simulink model "Mains"  (Simulink 8.7)
settings: Solver=ode23tb  SolverMode=SingleTasking  StartTime=0.0  StopTime=tfinal  FixedStep=dt  MaxStep=Ts/2  RelTol=1e-6  AbsTol=1e-6
values from neighbouring files (symbols this model uses):
  Dm = 0    [Para_Motor.m]
  Jm = 0.0532    [Para_Motor.m]
  Ld = 2.7e-3    (= 0.0027)    [Para_Motor.m]
  Lq = Ld    (= 0.0027)    [Para_Motor.m]
  Ofq = Ofpm*3/2*K_3T2    [Para_Motor.m]
  p = 4    [Para_Motor.m]
  Qm0 = 0    [Para_Motor.m]
  Ra = 0.145    [Para_Motor.m]
undefined symbols (not defined in the file or in its folder): DiscIntNeverNeededParam, fw_downlimit, fw_ki, fw_kp, fw_uplimit, Igbt_max, Jo, K_2T3, K_3T2, Kaff, Kid, Kiq, Kpp, Kpv, KTo, Kvff, Ldo, Lqo, magnitude, Ofqo, Svm, Tid, Tiq, Tiv, Tload, Trmax, Tsf, Tsi, Tsp, Tsr, Tsv, Udm, Uidm, Uiqm, Upm, Uqm, Urm, v_sat_fw, VoltCom_sw, Wrmax
undefined symbols (not defined in the file): T_cic_r, T_lpf_fw_ud, T_lpf_fw_uq, T_lpf_r, Tf
libraries: simulink x2
CloseFcn:
  | ;slview('closediagram',bdroot);
settings Model: Creator=zwn  LastModifiedBy=googol
settings SolverCC: ZeroCrossControl=DisableAll
settings DataIOCC: LimitDataPoints=off  SignalLoggingSaveFormat=ModelDataLogs  SaveOutput=off  SaveTime=off
settings OptimizationCC: BooleanDataType=off  ExpressionDepthLimit=2147483647  InitFltsAndDblsToZero=on
settings DebuggingCC: SaveWithParameterizedLinksMsg=none  SignalResolutionControl=TryResolveAllWithWarning  MultiTaskDSMMsg=warning  MultiTaskCondExecSysMsg=none  FcnCallInpInsideContextMsg=UseLocalSettings  UnconnectedInputMsg=none  UnconnectedOutputMsg=none  UnconnectedLineMsg=none  StateNameClashWarn=warning
settings HardwareCC: TargetUnknown=on
settings RTWCC: TemplateMakefile=grt.tmf
settings GRTTargetCC: TargetFcnLib=ansi_tfl_tmw.mat  ModelReferenceCompliant=off  CombineOutputUpdateFcns=off  MatFileLogging=off  GRTInterface=on

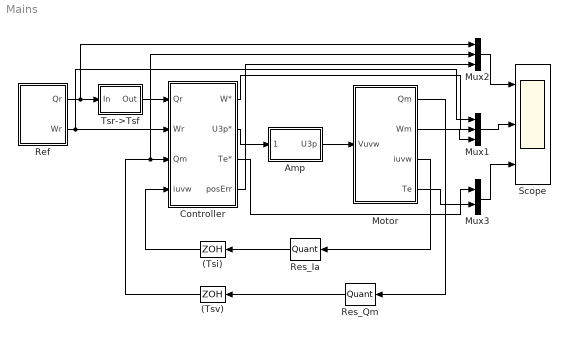
== system Mains ==
  (Tsi) : ZeroOrderHold  SampleTime=Tsi
  (Tsv) : ZeroOrderHold  SampleTime=Tsv
  Amp : Subsystem
  Controller : Subsystem
  Motor : Subsystem
  Mux1 : Mux  Inputs=3
  Mux2 : Mux  Inputs=3
  Mux3 : Mux  Inputs=2
  Ref : Subsystem
  Res_Ia : Quantizer  QuantizationInterval=Res_Ia
  Res_Qm : Quantizer  QuantizationInterval=Res_Qm
  Scope : Scope  NumInputPorts=3
  Tsr->Tsf : Subsystem
  wires:
  Motor/3(iuvw) -> Res_Ia/1
  (Tsi)/1 -> Controller/4(iuvw)
  Motor/1(Qm) -> Res_Qm/1
  (Tsv)/1 -> Controller/3(Qm), Mux2/2
  Mux1/1 -> Scope/2
  Res_Qm/1 -> (Tsv)/1
  Res_Ia/1 -> (Tsi)/1
  Ref/1(Qr) -> Tsr->Tsf/1(In), Mux2/1
  Tsr->Tsf/1(Out) -> Controller/1(Qr)
  Mux2/1 -> Scope/1
  Ref/2(Wr) -> Mux1/1, Controller/2(Wr)
  Mux3/1 -> Scope/3
  Motor/4(Te) -> Mux3/2
  Controller/3(Te*) -> Mux3/1
  Controller/2(U3p*) -> Amp/1(U3p*)
  Amp/1(U3p) -> Motor/1(Vuvw)
  Controller/4(posErr) -> Mux2/3
  Motor/2(Wm) -> Mux1/3
  Controller/1(W*) -> Mux1/2

== system Mains/Amp ==
  U3p* : Inport
  Constant2 : Constant  Value=[10 -5 -5]
  Manual Switch : ManualSwitch  CurrentSetting=0
  U3p : Outport
  wires:
  Constant2/1 -> Manual Switch/1
  Manual Switch/1 -> U3p/1
  U3p*/1 -> Manual Switch/2

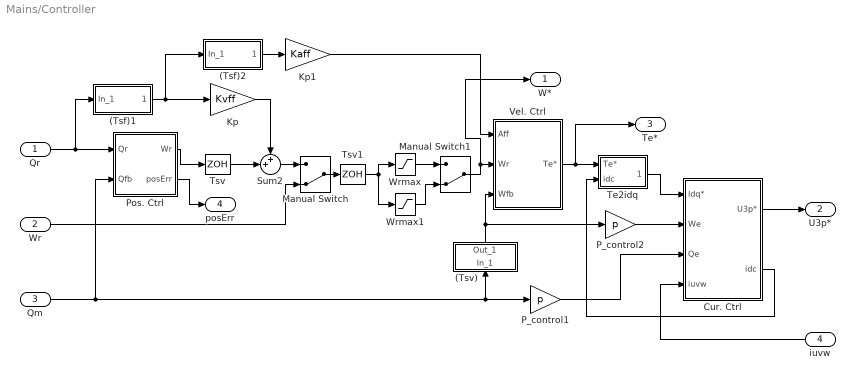
== system Mains/Controller ==
  Qr : Inport
  Wr : Inport  Port=2
  Qm : Inport  Port=3
  iuvw : Inport  Port=4
  (Tsf)1 : Subsystem  mask(Defference){Ts=Tsf, x0=0}
      mask prompts: Ts "Sample time Ts(s)"; x0 "Initial value x0"
      mask help: Enter expressions for a defference.
      mask Help: This block implements a defference. Unmask this block to see how it works. The defference term is implemented using a (1-z-1) block.
      mask Display: disp('(1-z-1)/Ts')
  (Tsf)2 : Subsystem  mask(Defference){Ts=Tsf, x0=0}
      mask prompts: Ts "Sample time Ts(s)"; x0 "Initial value x0"
      mask help: Enter expressions for a defference.
      mask Help: This block implements a defference. Unmask this block to see how it works. The defference term is implemented using a (1-z-1) block.
      mask Display: disp('(1-z-1)/Ts')
  (Tsv) : Subsystem  mask(Defference){Ts=Tsv, x0=Qm0}
      mask prompts: Ts "Sample time Ts(s)"; x0 "Initial value x0"
      mask help: Enter expressions for a defference.
      mask Help: This block implements a defference. Unmask this block to see how it works. The defference term is implemented using a (1-z-1) block.
      mask Display: disp('(1-z-1)/Ts')
  Cur. Ctrl : Subsystem
  Kp : Gain  Gain=Kvff  SaturateOnIntegerOverflow=on  OutDataTypeStr=Inherit: Same as input  ParamDataTypeStr=Inherit: Same as input
  Kp1 : Gain  Gain=Kaff  SaturateOnIntegerOverflow=on  OutDataTypeStr=Inherit: Same as input  ParamDataTypeStr=Inherit: Same as input
  Manual Switch : ManualSwitch  CurrentSetting=0
  Manual Switch1 : ManualSwitch  CurrentSetting=0
  P_control1 : Gain  Gain=p  SaturateOnIntegerOverflow=on  OutDataTypeStr=Inherit: Same as input  ParamDataTypeStr=Inherit: Same as input
  P_control2 : Gain  Gain=p  SaturateOnIntegerOverflow=on  OutDataTypeStr=Inherit: Same as input  ParamDataTypeStr=Inherit: Same as input
  Pos. Ctrl : Subsystem
  Sum2 : Sum  Inputs=++|  SampleTime=Tsp  SaturateOnIntegerOverflow=on  InputSameDT=on  OutDataTypeStr=Inherit: Same as first input
  Te2idq : Subsystem
  Tsv : ZeroOrderHold  SampleTime=Tsv
  Tsv1 : ZeroOrderHold  SampleTime=Tsv
  Vel. Ctrl : Subsystem
  Wrmax : Saturate  UpperLimit=Wrmax  LowerLimit=-Wrmax
  Wrmax1 : Saturate  UpperLimit=3*Wrmax  LowerLimit=-3*Wrmax
  W* : Outport
  U3p* : Outport  Port=2
  Te* : Outport  Port=3  InitialOutput=0
  posErr : Outport  Port=4
  wires:
  Qm/1 -> P_control1/1, (Tsv)/1(In_1), Pos. Ctrl/2(Qfb)
  P_control2/1 -> Cur. Ctrl/2(We)
  Vel. Ctrl/1(Te*) -> Te2idq/1(Te*), Te*/1
  Te2idq/1(Idq*) -> Cur. Ctrl/1(Idq*)
  (Tsv)/1(Out_1) -> Vel. Ctrl/3(Wfb), P_control2/1
  Cur. Ctrl/1(U3p*) -> U3p*/1
  P_control1/1 -> Cur. Ctrl/3(Qe)
  iuvw/1 -> Cur. Ctrl/4(iuvw)
  Pos. Ctrl/1(Wr) -> Tsv/1
  Qr/1 -> Pos. Ctrl/1(Qr), (Tsf)1/1(In_1)
  Tsv/1 -> Sum2/2
  (Tsf)1/1(Out_1) -> Kp/1, (Tsf)2/1(In_1)
  Kp/1 -> Sum2/1
  (Tsf)2/1(Out_1) -> Kp1/1
  Kp1/1 -> Vel. Ctrl/1(Aff)
  Sum2/1 -> Manual Switch/1
  Manual Switch/1 -> Tsv1/1
  Wr/1 -> Manual Switch/2
  Pos. Ctrl/2(posErr) -> posErr/1
  Cur. Ctrl/2(idc) -> Te2idq/2(idc)
  Wrmax/1 -> Manual Switch1/1
  Manual Switch1/1 -> W*/1, Vel. Ctrl/2(Wr)
  Wrmax1/1 -> Manual Switch1/2
  Tsv1/1 -> Wrmax/1, Wrmax1/1

== system Mains/Motor ==
  Vuvw : Inport
  Elec : Subsystem
  Mech : Subsystem
  Qm : Outport  InitialOutput=0
  Wm : Outport  Port=2  InitialOutput=0
  iuvw : Outport  Port=3  InitialOutput=0
  Te : Outport  Port=4  InitialOutput=0
  wires:
  Mech/2(Qm) -> Qm/1, Elec/3(Qm)
  Mech/1(Wm) -> Wm/1, Elec/2(Wm)
  Elec/1(iuvw) -> iuvw/1
  Elec/2(Te) -> Mech/1(Te), Te/1
  Vuvw/1 -> Elec/1(Vuvw)

== system Mains/Ref ==
  (T_cic_r,Tsr) : Subsystem  mask{n=round(T_cic_r/Tsr), Ts=Tsr}
      mask prompts: n "Steps"; Ts "Sampling time(s)"
      mask Display: disp('(1-z-n)/n(1-z-1)')
  1/s(Tsr) : DiscreteIntegrator  SampleTime=Tsr  UpperSaturationLimit=Trmax  LowerSaturationLimit=-Trmax  ICPrevOutput=DiscIntNeverNeededParam  ICPrevScaledInput=DiscIntNeverNeededParam
  Manual Switch : ManualSwitch
  Manual Switch1 : ManualSwitch
  Tf(Ts) : Subsystem  mask{Ts=Tsr, TL=T_lpf_r}
      mask prompts: Ts "Ts(s)"; TL "TL(s)"
      mask Display: disp('1/(1+TLs)')
  Wrr(rad/s) (Tsr) : FromWorkspace  VariableName=[twr,Wrr]  SampleTime=Tsr
  Qr : Outport
  Wr : Outport  Port=2
  wires:
  Wrr(rad/s) (Tsr)/1 -> (T_cic_r,Tsr)/1(In1), Manual Switch1/2, Tf(Ts)/1(In1)
  1/s(Tsr)/1 -> Qr/1
  Manual Switch/1 -> Wr/1, 1/s(Tsr)/1
  Tf(Ts)/1(Out1) -> Manual Switch/2
  Manual Switch1/1 -> Manual Switch/1
  (T_cic_r,Tsr)/1(Out1) -> Manual Switch1/1

== system Mains/Tsr->Tsf ==
  In : Inport
  Tsf : ZeroOrderHold  SampleTime=Tsf
  Tsr/Tsp(Tsf) : Subsystem  mask{n=round(Tsr/Tsf), Ts=Tsf}
      mask prompts: n "Sample number"; Ts "Sampling time(s)"
      mask Display: disp('CIC')
  Out : Outport
  wires:
  Tsf/1 -> Tsr/Tsp(Tsf)/1(In)
  In/1 -> Tsf/1
  Tsr/Tsp(Tsf)/1(Out) -> Out/1

== system Mains/Controller/(Tsf)1 ==
  In_1 : Inport
  Sum3 : Sum  Inputs=|+-  SaturateOnIntegerOverflow=on  InputSameDT=on  OutDataTypeStr=Inherit: Same as first input
  Ts(x0) : UnitDelay  InitialCondition=x0  SampleTime=Ts
  gear2 : Gain  Gain=1/Ts  SaturateOnIntegerOverflow=on  OutDataTypeStr=Inherit: Same as input  ParamDataTypeStr=Inherit: Same as input
  Out_1 : Outport  InitialOutput=0
  wires:
  In_1/1 -> Ts(x0)/1, Sum3/1
  Ts(x0)/1 -> Sum3/2
  Sum3/1 -> gear2/1
  gear2/1 -> Out_1/1

== system Mains/Controller/(Tsf)2 ==
  In_1 : Inport
  Sum3 : Sum  Inputs=|+-  SaturateOnIntegerOverflow=on  InputSameDT=on  OutDataTypeStr=Inherit: Same as first input
  Ts(x0) : UnitDelay  InitialCondition=x0  SampleTime=Ts
  gear2 : Gain  Gain=1/Ts  SaturateOnIntegerOverflow=on  OutDataTypeStr=Inherit: Same as input  ParamDataTypeStr=Inherit: Same as input
  Out_1 : Outport  InitialOutput=0
  wires:
  gear2/1 -> Out_1/1
  Sum3/1 -> gear2/1
  Ts(x0)/1 -> Sum3/2
  In_1/1 -> Sum3/1, Ts(x0)/1

== system Mains/Controller/(Tsv) ==
  In_1 : Inport
  Sum3 : Sum  Inputs=|+-  SaturateOnIntegerOverflow=on  InputSameDT=on  OutDataTypeStr=Inherit: Same as first input
  Ts(x0) : UnitDelay  InitialCondition=x0  SampleTime=Ts
  gear2 : Gain  Gain=1/Ts  SaturateOnIntegerOverflow=on  OutDataTypeStr=Inherit: Same as input  ParamDataTypeStr=Inherit: Same as input
  Out_1 : Outport  InitialOutput=0
  wires:
  gear2/1 -> Out_1/1
  Sum3/1 -> gear2/1
  Ts(x0)/1 -> Sum3/2
  In_1/1 -> Sum3/1, Ts(x0)/1

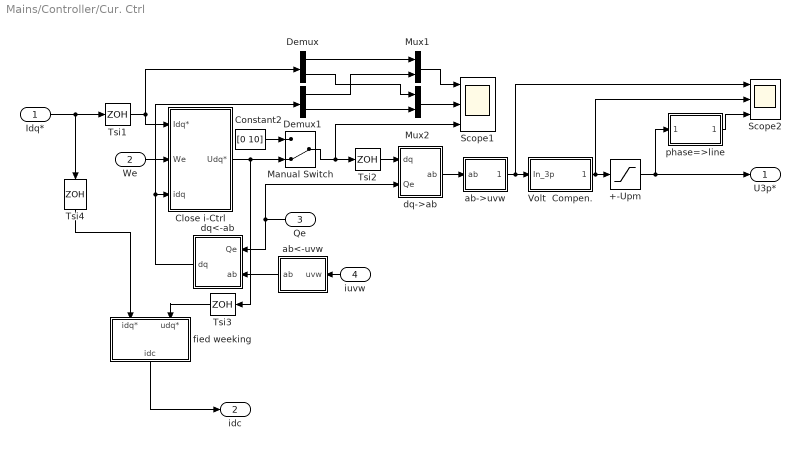
== system Mains/Controller/Cur. Ctrl ==
  Idq* : Inport
  We : Inport  Port=2
  Qe : Inport  Port=3
  iuvw : Inport  Port=4
  +-Upm : Saturate  UpperLimit=Upm  LowerLimit=-Upm
  Close i-Ctrl : Subsystem  TreatAsAtomicUnit=on
  Constant2 : Constant  Value=[0 10]
  Demux : Demux  Outputs=2
  Demux1 : Demux  Outputs=2
  Manual Switch : ManualSwitch  CurrentSetting=0
  Mux1 : Mux  Inputs=2
  Mux2 : Mux  Inputs=2
  Scope1 : Scope  NumInputPorts=3
  Scope2 : Scope  NumInputPorts=3
  Tsi{1..4} (4 alike) : ZeroOrderHold  SampleTime=Tsi
  Volt  Compen. : Subsystem
  ab->uvw : Subsystem
  ab<-uvw : Subsystem  TreatAsAtomicUnit=on
  dq->ab : Subsystem
  dq<-ab : Subsystem  TreatAsAtomicUnit=on
  fied weeking : Subsystem
  phase=>line : Subsystem
  U3p* : Outport
  idc : Outport  Port=2
  wires:
  Volt  Compen./1(Out_3p) -> +-Upm/1, Scope2/2
  dq->ab/1(ab) -> ab->uvw/1(ab)
  ab<-uvw/1(ab) -> dq<-ab/2(ab)
  iuvw/1 -> ab<-uvw/1(uvw)
  ab->uvw/1(uvw) -> Volt  Compen./1(In_3p), Scope2/1
  dq<-ab/1(dq) -> Close i-Ctrl/3(idq), Demux1/1
  Close i-Ctrl/1(Udq*) -> Tsi3/1, Manual Switch/2
  Manual Switch/1 -> Scope1/3, Tsi2/1
  Constant2/1 -> Manual Switch/1
  Qe/1 -> dq<-ab/1(Qe), dq->ab/2(Qe)
  Tsi1/1 -> Demux/1, Close i-Ctrl/1(Idq*)
  Mux1/1 -> Scope1/1
  Mux2/1 -> Scope1/2
  Demux/1 -> Mux1/1
  Demux1/1 -> Mux1/2
  Demux/2 -> Mux2/1
  Demux1/2 -> Mux2/2
  +-Upm/1 -> U3p*/1, phase=>line/1(U3p*)
  Idq*/1 -> Tsi4/1, Tsi1/1
  We/1 -> Close i-Ctrl/2(We)
  Tsi2/1 -> dq->ab/1(dq)
  phase=>line/1(U3l*) -> Scope2/3
  fied weeking/1(idc) -> idc/1
  Tsi3/1 -> fied weeking/2(udq*)
  Tsi4/1 -> fied weeking/1(idq*)

== system Mains/Controller/Pos. Ctrl ==
  Qr : Inport
  Qfb : Inport  Port=2
  Kp : Gain  Gain=Kpp  SaturateOnIntegerOverflow=on  OutDataTypeStr=Inherit: Same as input  ParamDataTypeStr=Inherit: Same as input
  Sum2 : Sum  Inputs=|+-  SampleTime=Tsp  SaturateOnIntegerOverflow=on  InputSameDT=on  OutDataTypeStr=Inherit: Same as first input
  Wr : Outport
  posErr : Outport  Port=2
  wires:
  Sum2/1 -> posErr/1, Kp/1
  Qfb/1 -> Sum2/2
  Qr/1 -> Sum2/1
  Kp/1 -> Wr/1

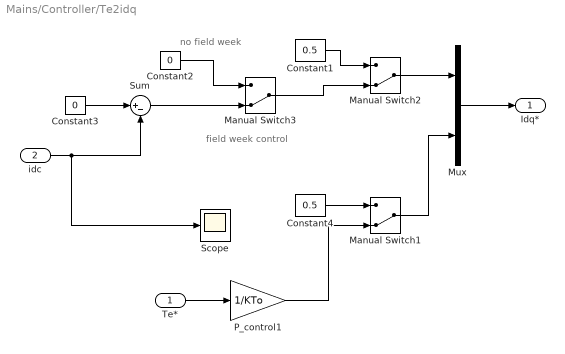
== system Mains/Controller/Te2idq ==
  note: field week control
  note: no field week
  Te* : Inport
  idc : Inport  Port=2
  Constant1 : Constant  Value=0.5
  Constant2 : Constant  Value=0
  Constant3 : Constant  Value=0
  Constant4 : Constant  Value=0.5
  Manual Switch1 : ManualSwitch  CurrentSetting=0
  Manual Switch2 : ManualSwitch  CurrentSetting=0
  Manual Switch3 : ManualSwitch  CurrentSetting=0
  Mux : Mux  Inputs=2
  P_control1 : Gain  Gain=1/KTo  SaturateOnIntegerOverflow=on  OutDataTypeStr=Inherit: Same as input  ParamDataTypeStr=Inherit: Same as input
  Scope : Scope
  Sum : Sum  Inputs=|+-
  Idq* : Outport
  wires:
  Te*/1 -> P_control1/1
  P_control1/1 -> Manual Switch1/2
  Constant1/1 -> Manual Switch2/1
  Manual Switch2/1 -> Mux/1
  Manual Switch1/1 -> Mux/2
  Mux/1 -> Idq*/1
  idc/1 -> Scope/1, Sum/2
  Constant3/1 -> Sum/1
  Sum/1 -> Manual Switch3/2
  Manual Switch3/1 -> Manual Switch2/2
  Constant2/1 -> Manual Switch3/1
  Constant4/1 -> Manual Switch1/1

== system Mains/Controller/Vel. Ctrl ==
  Aff : Inport
  Wr : Inport  Port=2
  Wfb : Inport  Port=3
  1/Ti : Gain  Gain=1/Tiv  SaturateOnIntegerOverflow=on  OutDataTypeStr=Inherit: Same as input  ParamDataTypeStr=Inherit: Same as input
  1/s : DiscreteIntegrator  SampleTime=Tsv  LimitOutput=on  UpperSaturationLimit=Svm  LowerSaturationLimit=-Svm  ICPrevOutput=DiscIntNeverNeededParam  ICPrevScaledInput=DiscIntNeverNeededParam
  P_control : Gain  Gain=Kpv  SaturateOnIntegerOverflow=on  OutDataTypeStr=Inherit: Same as input  ParamDataTypeStr=Inherit: Same as input
  P_control2 : Gain  Gain=Jo  SaturateOnIntegerOverflow=on  OutDataTypeStr=Inherit: Same as input  ParamDataTypeStr=Inherit: Same as input
  Sum : Sum  Inputs=+|+|+  SampleTime=Tsv  SaturateOnIntegerOverflow=on  InputSameDT=on  OutDataTypeStr=Inherit: Same as first input
  Sum1 : Sum  Inputs=|+-  SampleTime=Tsv  SaturateOnIntegerOverflow=on  InputSameDT=on  OutDataTypeStr=Inherit: Same as first input
  Tf(Ts) : Subsystem  mask{Ts=Tsv, TL=Tf}
      mask prompts: Ts "Ts(s)"; TL "TL(s)"
      mask Display: disp('1/(1+TLs)')
  Trmax : Saturate  UpperLimit=Trmax  LowerLimit=-Trmax
  Te* : Outport  InitialOutput=0
  wires:
  Sum/1 -> P_control2/1
  Sum1/1 -> P_control/1
  Wr/1 -> Sum1/1
  Wfb/1 -> Sum1/2
  Trmax/1 -> Tf(Ts)/1(In1)
  1/Ti/1 -> 1/s/1
  P_control/1 -> 1/Ti/1, Sum/3
  1/s/1 -> Sum/2
  Tf(Ts)/1(Out1) -> Te*/1
  P_control2/1 -> Trmax/1
  Aff/1 -> Sum/1

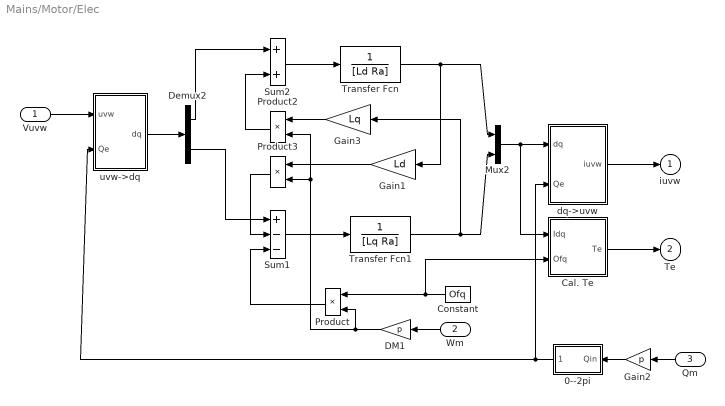
== system Mains/Motor/Elec ==
  Vuvw : Inport
  Wm : Inport  Port=2
  Qm : Inport  Port=3
  0--2pi : Subsystem
  Cal. Te : Subsystem
  Constant : Constant  Value=Ofq
  DM1 : Gain  Gain=p  SaturateOnIntegerOverflow=on  OutDataTypeStr=Inherit: Same as input  ParamDataTypeStr=Inherit: Same as input
  Demux2 : Demux  Outputs=2
  Gain1 : Gain  Gain=Ld  SaturateOnIntegerOverflow=on  OutDataTypeStr=Inherit: Same as input  ParamDataTypeStr=Inherit: Same as input
  Gain2 : Gain  Gain=p  SaturateOnIntegerOverflow=on  OutDataTypeStr=Inherit: Same as input  ParamDataTypeStr=Inherit: Same as input
  Gain3 : Gain  Gain=Lq  SaturateOnIntegerOverflow=on  OutDataTypeStr=Inherit: Same as input  ParamDataTypeStr=Inherit: Same as input
  Mux2 : Mux  Inputs=2
  Product : Product  SaturateOnIntegerOverflow=on  RndMeth=Zero  InputSameDT=on  OutDataTypeStr=Inherit: Same as first input
  Product2 : Product  SaturateOnIntegerOverflow=on  RndMeth=Zero  InputSameDT=on  OutDataTypeStr=Inherit: Same as first input
  Product3 : Product  SaturateOnIntegerOverflow=on  RndMeth=Zero  InputSameDT=on  OutDataTypeStr=Inherit: Same as first input
  Sum1 : Sum  Inputs=+--  SaturateOnIntegerOverflow=on  InputSameDT=on  OutDataTypeStr=Inherit: Same as first input
  Sum2 : Sum  SaturateOnIntegerOverflow=on  InputSameDT=on  OutDataTypeStr=Inherit: Same as first input
  Transfer Fcn : TransferFcn  Denominator=[Ld Ra]
  Transfer Fcn1 : TransferFcn  Denominator=[Lq Ra]
  dq->uvw : Subsystem
  uvw->dq : Subsystem
  iuvw : Outport  InitialOutput=0
  Te : Outport  Port=2  InitialOutput=0
  wires:
  0--2pi/1(Qout) -> dq->uvw/2(Qe), uvw->dq/2(Qe)
  Product/1 -> Sum1/3
  Constant/1 -> Product/1, Cal. Te/2(Ofq)
  Mux2/1 -> dq->uvw/1(dq), Cal. Te/1(Idq)
  dq->uvw/1(iuvw) -> iuvw/1
  DM1/1 -> Product/2, Product3/2, Product2/2
  Wm/1 -> DM1/1
  Product2/1 -> Sum2/2
  Product3/1 -> Sum1/2
  Gain1/1 -> Product3/1
  Gain3/1 -> Product2/1
  Demux2/2 -> Sum1/1
  Transfer Fcn/1 -> Mux2/1, Gain1/1
  Transfer Fcn1/1 -> Mux2/2, Gain3/1
  Sum1/1 -> Transfer Fcn1/1
  Demux2/1 -> Sum2/1
  uvw->dq/1(dq) -> Demux2/1
  Sum2/1 -> Transfer Fcn/1
  Qm/1 -> Gain2/1
  Gain2/1 -> 0--2pi/1(Qin)
  Vuvw/1 -> uvw->dq/1(uvw)
  Cal. Te/1(Te) -> Te/1

== system Mains/Motor/Mech ==
  Te : Inport
  1/JM : Gain  Gain=1/Jm  SaturateOnIntegerOverflow=on  OutDataTypeStr=Inherit: Same as input  ParamDataTypeStr=Inherit: Same as input
  Constant2 : Constant  Value=Tload
  DM : Gain  Gain=Dm  SaturateOnIntegerOverflow=on  OutDataTypeStr=Inherit: Same as input  ParamDataTypeStr=Inherit: Same as input
  Qm0 : Integrator  InitialCondition=Qm0
  Sum1 : Sum  Inputs=-|+|-  SaturateOnIntegerOverflow=on  InputSameDT=on  OutDataTypeStr=Inherit: Same as first input
  velocity4 : Integrator
  Wm : Outport  InitialOutput=0
  Qm : Outport  Port=2  InitialOutput=0
  wires:
  1/JM/1 -> velocity4/1
  Qm0/1 -> Qm/1
  velocity4/1 -> Qm0/1, DM/1, Wm/1
  Te/1 -> Sum1/2
  Sum1/1 -> 1/JM/1
  Constant2/1 -> Sum1/3
  DM/1 -> Sum1/1

== system Mains/Ref/(T_cic_r,Tsr) ==
  In1 : Inport
  (1/z)^n : DiscreteTransferFcn  Denominator=[1 zeros(1,n)]  SampleTime=Ts
  1/z(Ts) : UnitDelay  SampleTime=Ts
  Sum3 : Sum  Inputs=-+|  SaturateOnIntegerOverflow=on  InputSameDT=on  OutDataTypeStr=Inherit: Same as first input
  Sum4 : Sum  Inputs=|++  SaturateOnIntegerOverflow=on  InputSameDT=on  OutDataTypeStr=Inherit: Same as first input
  pMum : Gain  Gain=1/n  SaturateOnIntegerOverflow=on  OutDataTypeStr=Inherit: Same as input  ParamDataTypeStr=Inherit: Same as input
  Out1 : Outport
  wires:
  pMum/1 -> Sum4/1
  Sum4/1 -> 1/z(Ts)/1, Out1/1
  1/z(Ts)/1 -> Sum4/2
  Sum3/1 -> pMum/1
  (1/z)^n/1 -> Sum3/1
  In1/1 -> (1/z)^n/1, Sum3/2

== system Mains/Ref/Tf(Ts) ==
  In1 : Inport
  LPF : DiscreteFilter  Numerator=[Ts/(Ts+TL)]  Denominator=[1 -(1-Ts/(Ts+TL))]  SampleTime=Ts
  Out1 : Outport
  wires:
  LPF/1 -> Out1/1
  In1/1 -> LPF/1

== system Mains/Tsr->Tsf/Tsr/Tsp(Tsf) ==
  In : Inport
  (1/z)^n : DiscreteTransferFcn  Denominator=[1 zeros(1,n)]  SampleTime=Ts
  1/z(Ts) : UnitDelay  SampleTime=Ts
  Sum3 : Sum  Inputs=-+|  SampleTime=Ts  SaturateOnIntegerOverflow=on  InputSameDT=on  OutDataTypeStr=Inherit: Same as first input
  Sum4 : Sum  Inputs=|++  SaturateOnIntegerOverflow=on  InputSameDT=on  OutDataTypeStr=Inherit: Same as first input
  pMum : Gain  Gain=1/n  SaturateOnIntegerOverflow=on  OutDataTypeStr=Inherit: Same as input  ParamDataTypeStr=Inherit: Same as input
  Out : Outport
  wires:
  In/1 -> Sum3/2, (1/z)^n/1
  (1/z)^n/1 -> Sum3/1
  Sum3/1 -> Sum4/1
  1/z(Ts)/1 -> Sum4/2
  Sum4/1 -> 1/z(Ts)/1, pMum/1
  pMum/1 -> Out/1

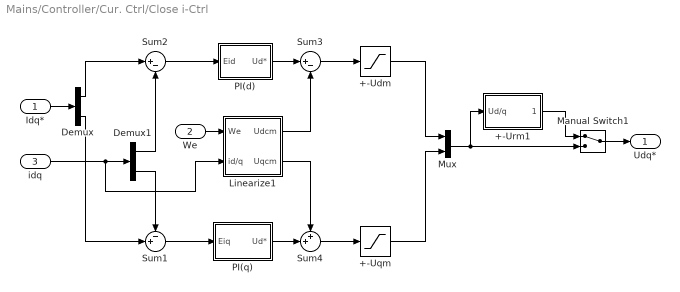
== system Mains/Controller/Cur. Ctrl/Close i-Ctrl ==
  Idq* : Inport
  We : Inport  Port=2
  idq : Inport  Port=3
  +-Udm : Saturate  UpperLimit=Udm  LowerLimit=-Udm
  +-Uqm : Saturate  UpperLimit=Uqm  LowerLimit=-Uqm
  +-Urm1 : Subsystem
  Demux : Demux  Outputs=2
  Demux1 : Demux  Outputs=2
  Linearize1 : Subsystem  TreatAsAtomicUnit=on
  Manual Switch1 : ManualSwitch
  Mux : Mux  Inputs=2
  PI(d) : Subsystem
  PI(q) : Subsystem
  Sum1 : Sum  Inputs=-+|  SaturateOnIntegerOverflow=on  InputSameDT=on  OutDataTypeStr=Inherit: Same as first input
  Sum2 : Sum  Inputs=|+-  SaturateOnIntegerOverflow=on  InputSameDT=on  OutDataTypeStr=Inherit: Same as first input
  Sum3 : Sum  Inputs=|+-  SaturateOnIntegerOverflow=on  InputSameDT=on  OutDataTypeStr=Inherit: Same as first input
  Sum4 : Sum  Inputs=++|  SaturateOnIntegerOverflow=on  InputSameDT=on  OutDataTypeStr=Inherit: Same as first input
  Udq* : Outport
  wires:
  idq/1 -> Linearize1/2(id/q), Demux1/1
  We/1 -> Linearize1/1(We)
  Sum4/1 -> +-Uqm/1
  Sum3/1 -> +-Udm/1
  PI(q)/1(Ud*) -> Sum4/2
  Demux1/1 -> Sum2/2
  Demux1/2 -> Sum1/1
  Sum2/1 -> PI(d)/1(Eid)
  PI(d)/1(Ud*) -> Sum3/1
  Sum1/1 -> PI(q)/1(Eiq)
  +-Udm/1 -> Mux/1
  +-Uqm/1 -> Mux/2
  Demux/1 -> Sum2/1
  Idq*/1 -> Demux/1
  Demux/2 -> Sum1/2
  Linearize1/1(Udcm) -> Sum3/2
  Linearize1/2(Uqcm) -> Sum4/1
  Manual Switch1/1 -> Udq*/1
  Mux/1 -> Manual Switch1/2, +-Urm1/1(Ud/q)
  +-Urm1/1(Ud/qO) -> Manual Switch1/1

== system Mains/Controller/Cur. Ctrl/Volt  Compen. ==
  In_3p : Inport
  Constant : Constant  Value=VoltCom_sw
  Constant1 : Constant  Value=0
  Multiport Switch : MultiPortSwitch  SampleTime=Tsi  SaturateOnIntegerOverflow=on  InputSameDT=on
  Sum3 : Sum  SaturateOnIntegerOverflow=on  InputSameDT=on  OutDataTypeStr=Inherit: Same as first input
  Volt Compen 1 : Subsystem
  Volt Compen 2 : Subsystem
  Out_3p : Outport
  wires:
  In_3p/1 -> Volt Compen 1/1(Uuvw), Volt Compen 2/1(Uuvw), Sum3/1
  Multiport Switch/1 -> Sum3/2
  Constant1/1 -> Multiport Switch/4
  Constant/1 -> Multiport Switch/1
  Volt Compen 2/1(Uh2) -> Multiport Switch/3
  Volt Compen 1/1(Uh1) -> Multiport Switch/2
  Sum3/1 -> Out_3p/1

== system Mains/Controller/Cur. Ctrl/ab->uvw ==
  ab : Inport
  Constant1 : Constant  Value=[-1/2 sqrt(3)/2]  SampleTime=Tsi
  Constant2 : Constant  Value=[1 0]  SampleTime=Tsi
  Constant3 : Constant  Value=[-1/2 -sqrt(3)/2]  SampleTime=Tsi
  Dot Product : DotProduct  InputSameDT=on  OutDataTypeStr=Inherit: Inherit via internal rule
  Dot Product1 : DotProduct  InputSameDT=on  OutDataTypeStr=Inherit: Inherit via internal rule
  Dot Product2 : DotProduct  InputSameDT=on  OutDataTypeStr=Inherit: Inherit via internal rule
  Gain5 : Gain  Gain=K_2T3  SaturateOnIntegerOverflow=on  OutDataTypeStr=Inherit: Same as input  ParamDataTypeStr=Inherit: Same as input
  Mux1 : Mux  Inputs=3
  uvw : Outport  InitialOutput=0
  wires:
  Dot Product1/1 -> Mux1/2
  Dot Product/1 -> Mux1/1
  Constant2/1 -> Dot Product/2
  Constant1/1 -> Dot Product1/2
  ab/1 -> Dot Product/1, Dot Product1/1, Dot Product2/1
  Mux1/1 -> Gain5/1
  Constant3/1 -> Dot Product2/2
  Dot Product2/1 -> Mux1/3
  Gain5/1 -> uvw/1

== system Mains/Controller/Cur. Ctrl/ab<-uvw ==
  uvw : Inport
  Constant1 : Constant  Value=[0 1 -1]*sqrt(3)/2  SampleTime=Tsi
  Constant2 : Constant  Value=[1 -0.5 -0.5]  SampleTime=Tsi
  Dot Product : DotProduct  InputSameDT=on  OutDataTypeStr=Inherit: Inherit via internal rule
  Dot Product1 : DotProduct  InputSameDT=on  OutDataTypeStr=Inherit: Inherit via internal rule
  Gain5 : Gain  Gain=K_3T2  SaturateOnIntegerOverflow=on  OutDataTypeStr=Inherit: Same as input  ParamDataTypeStr=Inherit: Same as input
  Mux1 : Mux  Inputs=2
  ab : Outport  InitialOutput=0
  wires:
  Dot Product1/1 -> Mux1/2
  Constant1/1 -> Dot Product1/2
  Dot Product/1 -> Mux1/1
  uvw/1 -> Dot Product1/1, Dot Product/1
  Constant2/1 -> Dot Product/2
  Gain5/1 -> ab/1
  Mux1/1 -> Gain5/1

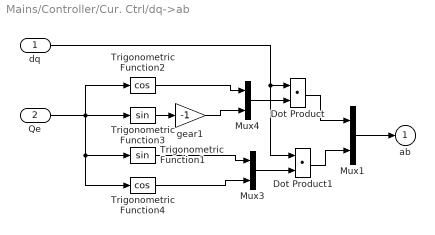
== system Mains/Controller/Cur. Ctrl/dq->ab ==
  dq : Inport
  Qe : Inport  Port=2
  Dot Product : DotProduct  InputSameDT=on  OutDataTypeStr=Inherit: Inherit via internal rule
  Dot Product1 : DotProduct  InputSameDT=on  OutDataTypeStr=Inherit: Inherit via internal rule
  Mux1 : Mux  Inputs=2
  Mux3 : Mux  Inputs=2
  Mux4 : Mux  Inputs=2
  Trigonometric Function1 : Trigonometry
  Trigonometric Function2 : Trigonometry  Operator=cos
  Trigonometric Function3 : Trigonometry
  Trigonometric Function4 : Trigonometry  Operator=cos
  gear1 : Gain  Gain=-1  SaturateOnIntegerOverflow=on  OutDataTypeStr=Inherit: Same as input  ParamDataTypeStr=Inherit: Same as input
  ab : Outport  InitialOutput=0
  wires:
  Mux1/1 -> ab/1
  dq/1 -> Dot Product/1, Dot Product1/1
  Qe/1 -> Trigonometric Function3/1, Trigonometric Function2/1, Trigonometric Function1/1, Trigonometric Function4/1
  Trigonometric Function1/1 -> Mux3/1
  Trigonometric Function4/1 -> Mux3/2
  Trigonometric Function2/1 -> Mux4/1
  Trigonometric Function3/1 -> gear1/1
  Mux3/1 -> Dot Product1/2
  Mux4/1 -> Dot Product/2
  Dot Product1/1 -> Mux1/2
  Dot Product/1 -> Mux1/1
  gear1/1 -> Mux4/2

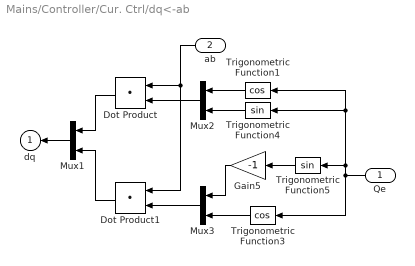
== system Mains/Controller/Cur. Ctrl/dq<-ab ==
  Qe : Inport
  ab : Inport  Port=2
  Dot Product : DotProduct  InputSameDT=on  OutDataTypeStr=Inherit: Inherit via internal rule
  Dot Product1 : DotProduct  InputSameDT=on  OutDataTypeStr=Inherit: Inherit via internal rule
  Gain5 : Gain  Gain=-1  SaturateOnIntegerOverflow=on  OutDataTypeStr=Inherit: Same as input  ParamDataTypeStr=Inherit: Same as input
  Mux1 : Mux  Inputs=2
  Mux2 : Mux  Inputs=2
  Mux3 : Mux  Inputs=2
  Trigonometric Function1 : Trigonometry  Operator=cos
  Trigonometric Function3 : Trigonometry  Operator=cos
  Trigonometric Function4 : Trigonometry
  Trigonometric Function5 : Trigonometry
  dq : Outport  InitialOutput=0
  wires:
  Dot Product1/1 -> Mux1/2
  Mux3/1 -> Dot Product1/2
  Dot Product/1 -> Mux1/1
  ab/1 -> Dot Product1/1, Dot Product/1
  Mux2/1 -> Dot Product/2
  Trigonometric Function1/1 -> Mux2/1
  Mux1/1 -> dq/1
  Trigonometric Function4/1 -> Mux2/2
  Trigonometric Function3/1 -> Mux3/2
  Trigonometric Function5/1 -> Gain5/1
  Qe/1 -> Trigonometric Function1/1, Trigonometric Function4/1, Trigonometric Function5/1, Trigonometric Function3/1
  Gain5/1 -> Mux3/1

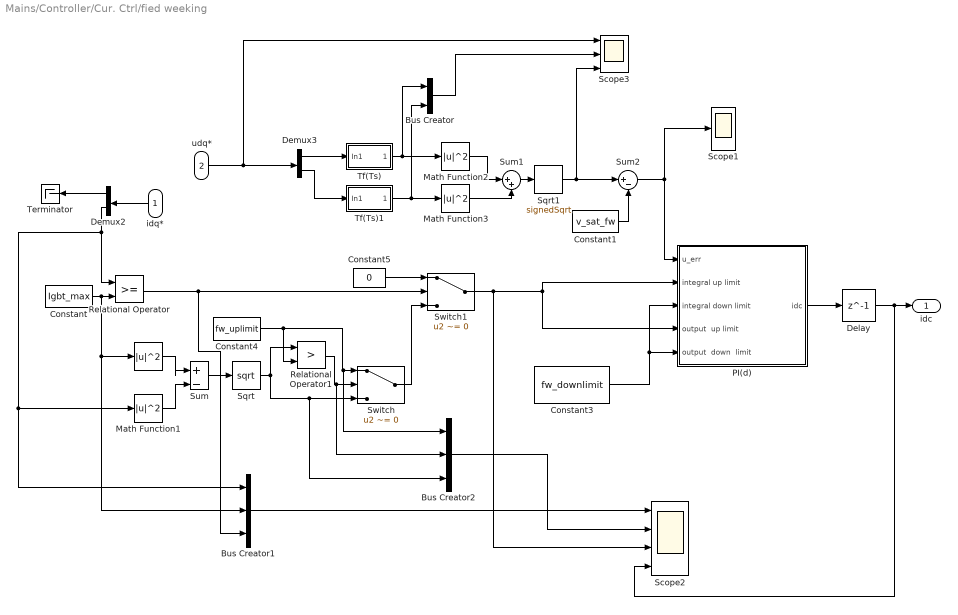
== system Mains/Controller/Cur. Ctrl/fied weeking ==
  idq* : Inport
  udq* : Inport  Port=2
  " " : Math  Operator=magnitude^2  SaturateOnIntegerOverflow=on
  Bus Creator : BusCreator  Inputs=2
  Bus Creator1 : BusCreator  Inputs=3
  Bus Creator2 : BusCreator  Inputs=3
  Constant : Constant  Value=Igbt_max
  Constant1 : Constant  Value=v_sat_fw
  Constant3 : Constant  Value=fw_downlimit
  Constant4 : Constant  Value=fw_uplimit
  Constant5 : Constant  Value=0
  Delay : Delay  DelayLength=1  SampleTime=Tsi
  Demux2 : Demux  Outputs=2
  Demux3 : Demux  Outputs=2
  Math Function1 : Math  Operator=magnitude^2  SaturateOnIntegerOverflow=on
  Math Function2 : Math  Operator=magnitude^2  OutputSignalType=real  SaturateOnIntegerOverflow=on
  Math Function3 : Math  Operator=magnitude^2  OutputSignalType=real  SaturateOnIntegerOverflow=on
  PI(d) : Subsystem
  Relational Operator : RelationalOperator  InputSameDT=on
  Relational Operator1 : RelationalOperator  Operator=>  InputSameDT=on
  Scope1 : Scope
  Scope2 : Scope  NumInputPorts=4
  Scope3 : Scope  NumInputPorts=3
  Sqrt : Sqrt  SaturateOnIntegerOverflow=on
  Sqrt1 : Sqrt  Operator=signedSqrt  OutputSignalType=real  SaturateOnIntegerOverflow=on
  Sum : Sum  Inputs=|+-
  Sum1 : Sum  Inputs=|++
  Sum2 : Sum  Inputs=|+-
  Switch : Switch  Criteria=u2 ~= 0
  Switch1 : Switch  Criteria=u2 ~= 0
  Terminator : Terminator
  Tf(Ts) : Subsystem  mask{Ts=Tsi, TL=T_lpf_fw_ud}
      mask prompts: Ts "Ts(s)"; TL "TL(s)"
      mask Display: disp('1/(1+TLs)')
  Tf(Ts)1 : Subsystem  mask{Ts=Tsi, TL=T_lpf_fw_uq}
      mask prompts: Ts "Ts(s)"; TL "TL(s)"
      mask Display: disp('1/(1+TLs)')
  idc : Outport
  wires:
  Demux2/2 -> Bus Creator1/1, Math Function1/1, Relational Operator/1
  Demux2/1 -> Terminator/1
  Relational Operator1/1 -> Bus Creator2/2, Switch/2
  Constant/1 -> Bus Creator1/2, " "/1, Relational Operator/2
  PI(d)/1(idc) -> Delay/1
  Switch/1 -> Switch1/3
  Constant5/1 -> Switch1/1
  Switch1/1 -> PI(d)/2(integral up limit), PI(d)/4(output  up limit), Scope2/3
  Tf(Ts)/1(Out1) -> Bus Creator/1, Math Function2/1
  Tf(Ts)1/1(Out1) -> Bus Creator/2, Math Function3/1
  Sum/1 -> Sqrt/1
  Constant3/1 -> PI(d)/3(integral down limit), PI(d)/5(output  down  limit)
  Relational Operator/1 -> Bus Creator1/3, Switch1/2
  " "/1 -> Sum/1
  Math Function1/1 -> Sum/2
  Constant1/1 -> Sum2/2
  Math Function3/1 -> Sum1/2
  udq*/1 -> Scope3/1, Demux3/1
  Sum1/1 -> Sqrt1/1
  Demux3/1 -> Tf(Ts)/1(In1)
  idq*/1 -> Demux2/1
  Demux3/2 -> Tf(Ts)1/1(In1)
  Math Function2/1 -> Sum1/1
  Sqrt1/1 -> Scope3/3, Sum2/1
  Constant4/1 -> Bus Creator2/1, Switch/1, Relational Operator1/2
  Sum2/1 -> Scope1/1, PI(d)/1(u_err)
  Sqrt/1 -> Relational Operator1/1, Bus Creator2/3, Switch/3
  Delay/1 -> Scope2/4, idc/1
  Bus Creator/1 -> Scope3/2
  Bus Creator1/1 -> Scope2/1
  Bus Creator2/1 -> Scope2/2

== system Mains/Controller/Cur. Ctrl/phase=>line ==
  U3p* : Inport
  Demux2 : Demux  Outputs=3
  Mux3 : Mux  Inputs=3
  Sum1 : Sum  Inputs=|+-  SaturateOnIntegerOverflow=on  InputSameDT=on  OutDataTypeStr=Inherit: Same as first input
  Sum2 : Sum  Inputs=|+-  SaturateOnIntegerOverflow=on  InputSameDT=on  OutDataTypeStr=Inherit: Same as first input
  Sum3 : Sum  Inputs=|+-  SaturateOnIntegerOverflow=on  InputSameDT=on  OutDataTypeStr=Inherit: Same as first input
  U3l* : Outport
  wires:
  Demux2/1 -> Sum2/1, Sum3/2
  Demux2/2 -> Sum1/1, Sum2/2
  Demux2/3 -> Sum3/1, Sum1/2
  Sum2/1 -> Mux3/1
  Sum1/1 -> Mux3/2
  Sum3/1 -> Mux3/3
  U3p*/1 -> Demux2/1
  Mux3/1 -> U3l*/1

== system Mains/Controller/Vel. Ctrl/Tf(Ts) ==
  In1 : Inport
  LPF : DiscreteFilter  Numerator=[Ts/(Ts+TL)]  Denominator=[1 -(1-Ts/(Ts+TL))]  SampleTime=Ts
  Out1 : Outport
  wires:
  LPF/1 -> Out1/1
  In1/1 -> LPF/1

== system Mains/Motor/Elec/0--2pi ==
  Qin : Inport
  Rounding Function : Rounding
  Sum2 : Sum  Inputs=|+-  SaturateOnIntegerOverflow=on  InputSameDT=on  OutDataTypeStr=Inherit: Same as first input
  ki1 : Gain  Gain=1/2/pi  SaturateOnIntegerOverflow=on  OutDataTypeStr=Inherit: Same as input  ParamDataTypeStr=Inherit: Same as input
  ki3 : Gain  Gain=2*pi  SaturateOnIntegerOverflow=on  OutDataTypeStr=Inherit: Same as input  ParamDataTypeStr=Inherit: Same as input
  Qout : Outport  InitialOutput=0
  wires:
  Qin/1 -> ki1/1
  ki3/1 -> Qout/1
  Sum2/1 -> ki3/1
  ki1/1 -> Sum2/1, Rounding Function/1
  Rounding Function/1 -> Sum2/2

== system Mains/Motor/Elec/Cal. Te ==
  Idq : Inport
  Ofq : Inport  Port=2
  DM : Gain  Gain=p  SaturateOnIntegerOverflow=on  OutDataTypeStr=Inherit: Same as input  ParamDataTypeStr=Inherit: Same as input
  Demux : Demux  Outputs=2
  Gain4 : Gain  Gain=Ld-Lq  SaturateOnIntegerOverflow=on  OutDataTypeStr=Inherit: Same as input  ParamDataTypeStr=Inherit: Same as input
  Product2 : Product  SaturateOnIntegerOverflow=on  RndMeth=Zero  InputSameDT=on  OutDataTypeStr=Inherit: Same as first input
  Sum2 : Sum  Inputs=++|  SampleTime=Tsp  SaturateOnIntegerOverflow=on  InputSameDT=on  OutDataTypeStr=Inherit: Same as first input
  Te : Outport
  wires:
  Idq/1 -> Demux/1
  Demux/1 -> Gain4/1
  DM/1 -> Te/1
  Gain4/1 -> Sum2/2
  Ofq/1 -> Sum2/1
  Sum2/1 -> Product2/1
  Demux/2 -> Product2/2
  Product2/1 -> DM/1

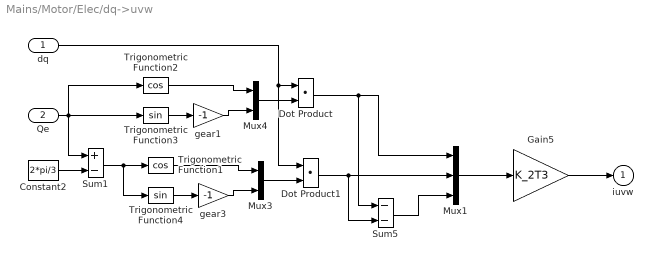
== system Mains/Motor/Elec/dq->uvw ==
  dq : Inport
  Qe : Inport  Port=2
  Constant2 : Constant  Value=2*pi/3
  Dot Product : DotProduct  InputSameDT=on  OutDataTypeStr=Inherit: Inherit via internal rule
  Dot Product1 : DotProduct  InputSameDT=on  OutDataTypeStr=Inherit: Inherit via internal rule
  Gain5 : Gain  Gain=K_2T3  SaturateOnIntegerOverflow=on  OutDataTypeStr=Inherit: Same as input  ParamDataTypeStr=Inherit: Same as input
  Mux1 : Mux  Inputs=3
  Mux3 : Mux  Inputs=2
  Mux4 : Mux  Inputs=2
  Sum1 : Sum  Inputs=+-  SaturateOnIntegerOverflow=on  InputSameDT=on  OutDataTypeStr=Inherit: Same as first input
  Sum5 : Sum  Inputs=--  SaturateOnIntegerOverflow=on  InputSameDT=on  OutDataTypeStr=Inherit: Same as first input
  Trigonometric Function1 : Trigonometry  Operator=cos
  Trigonometric Function2 : Trigonometry  Operator=cos
  Trigonometric Function3 : Trigonometry
  Trigonometric Function4 : Trigonometry
  gear1 : Gain  Gain=-1  SaturateOnIntegerOverflow=on  OutDataTypeStr=Inherit: Same as input  ParamDataTypeStr=Inherit: Same as input
  gear3 : Gain  Gain=-1  SaturateOnIntegerOverflow=on  OutDataTypeStr=Inherit: Same as input  ParamDataTypeStr=Inherit: Same as input
  iuvw : Outport  InitialOutput=0
  wires:
  Mux1/1 -> Gain5/1
  dq/1 -> Dot Product/1, Dot Product1/1
  Constant2/1 -> Sum1/2
  Qe/1 -> Sum1/1, Trigonometric Function3/1, Trigonometric Function2/1
  Sum1/1 -> Trigonometric Function1/1, Trigonometric Function4/1
  Trigonometric Function1/1 -> Mux3/1
  Trigonometric Function4/1 -> gear3/1
  gear3/1 -> Mux3/2
  Trigonometric Function2/1 -> Mux4/1
  Trigonometric Function3/1 -> gear1/1
  gear1/1 -> Mux4/2
  Mux3/1 -> Dot Product1/2
  Mux4/1 -> Dot Product/2
  Dot Product/1 -> Mux1/1, Sum5/1
  Dot Product1/1 -> Mux1/2, Sum5/2
  Sum5/1 -> Mux1/3
  Gain5/1 -> iuvw/1

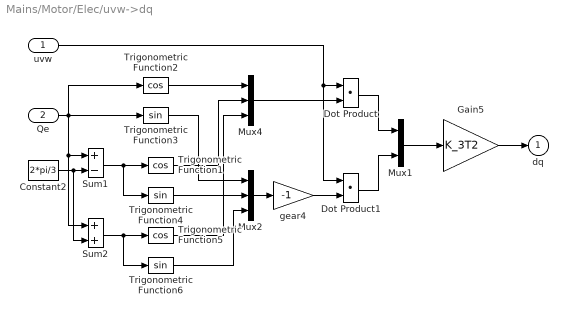
== system Mains/Motor/Elec/uvw->dq ==
  uvw : Inport
  Qe : Inport  Port=2
  Constant2 : Constant  Value=2*pi/3
  Dot Product : DotProduct  InputSameDT=on  OutDataTypeStr=Inherit: Inherit via internal rule
  Dot Product1 : DotProduct  InputSameDT=on  OutDataTypeStr=Inherit: Inherit via internal rule
  Gain5 : Gain  Gain=K_3T2  SaturateOnIntegerOverflow=on  OutDataTypeStr=Inherit: Same as input  ParamDataTypeStr=Inherit: Same as input
  Mux1 : Mux  Inputs=2
  Mux2 : Mux  Inputs=3
  Mux4 : Mux  Inputs=3
  Sum1 : Sum  Inputs=+-  SaturateOnIntegerOverflow=on  InputSameDT=on  OutDataTypeStr=Inherit: Same as first input
  Sum2 : Sum  SaturateOnIntegerOverflow=on  InputSameDT=on  OutDataTypeStr=Inherit: Same as first input
  Trigonometric Function1 : Trigonometry  Operator=cos
  Trigonometric Function2 : Trigonometry  Operator=cos
  Trigonometric Function3 : Trigonometry
  Trigonometric Function4 : Trigonometry
  Trigonometric Function5 : Trigonometry  Operator=cos
  Trigonometric Function6 : Trigonometry
  gear4 : Gain  Gain=-1  SaturateOnIntegerOverflow=on  OutDataTypeStr=Inherit: Same as input  ParamDataTypeStr=Inherit: Same as input
  dq : Outport  InitialOutput=0
  wires:
  gear4/1 -> Dot Product1/2
  Trigonometric Function5/1 -> Mux4/3
  Trigonometric Function1/1 -> Mux4/2
  Sum2/1 -> Trigonometric Function6/1, Trigonometric Function5/1
  Trigonometric Function6/1 -> Mux2/3
  Dot Product1/1 -> Mux1/2
  Dot Product/1 -> Mux1/1
  Mux4/1 -> Dot Product/2
  Mux2/1 -> gear4/1
  Trigonometric Function3/1 -> Mux2/1
  Trigonometric Function2/1 -> Mux4/1
  Trigonometric Function4/1 -> Mux2/2
  Sum1/1 -> Trigonometric Function4/1, Trigonometric Function1/1
  Qe/1 -> Sum2/1, Sum1/1, Trigonometric Function2/1, Trigonometric Function3/1
  Constant2/1 -> Sum2/2, Sum1/2
  uvw/1 -> Dot Product1/1, Dot Product/1
  Mux1/1 -> Gain5/1
  Gain5/1 -> dq/1

== system Mains/Controller/Cur. Ctrl/Close i-Ctrl/+-Urm1 ==
  Ud/q : Inport
  Constant : Constant  Value=Urm
  Recalculate : Subsystem  TreatAsAtomicUnit=on
  Relational Operator : RelationalOperator  Operator=>  InputSameDT=on
  Urm1 : Switch  Threshold=Urm  SaturateOnIntegerOverflow=on  InputSameDT=on
  sqrt(u(1)^2+u(2)^2) : Fcn  Expr=sqrt(u(1)^2+u(2)^2)
  Ud/qO : Outport
  wires:
  Ud/q/1 -> sqrt(u(1)^2+u(2)^2)/1, Urm1/3, Recalculate/1(Ud/q)
  sqrt(u(1)^2+u(2)^2)/1 -> Urm1/2, Recalculate/2(Ur), Relational Operator/1
  Urm1/1 -> Ud/qO/1
  Recalculate/1(Ud/qO) -> Urm1/1
  Constant/1 -> Relational Operator/2
  Relational Operator/1 -> Recalculate/Enable

== system Mains/Controller/Cur. Ctrl/Close i-Ctrl/Linearize1 ==
  We : Inport
  id/q : Inport  Port=2
  Demux : Demux  Outputs=2
  Product : Product  SaturateOnIntegerOverflow=on  RndMeth=Zero  InputSameDT=on  OutDataTypeStr=Inherit: Same as first input
  Product1 : Product  SaturateOnIntegerOverflow=on  RndMeth=Zero  InputSameDT=on  OutDataTypeStr=Inherit: Same as first input
  Sum7 : Sum  SaturateOnIntegerOverflow=on  InputSameDT=on  OutDataTypeStr=Inherit: Same as first input
  ki3 : Gain  Gain=Ofqo  SaturateOnIntegerOverflow=on  OutDataTypeStr=Inherit: Same as input  ParamDataTypeStr=Inherit: Same as input
  ki4 : Gain  Gain=Ldo  SaturateOnIntegerOverflow=on  OutDataTypeStr=Inherit: Same as input  ParamDataTypeStr=Inherit: Same as input
  ki5 : Gain  Gain=Lqo  SaturateOnIntegerOverflow=on  OutDataTypeStr=Inherit: Same as input  ParamDataTypeStr=Inherit: Same as input
  Udcm : Outport  InitialOutput=0
  Uqcm : Outport  Port=2  InitialOutput=0
  wires:
  Demux/2 -> ki5/1
  Demux/1 -> ki4/1
  id/q/1 -> Demux/1
  ki5/1 -> Product1/2
  Product1/1 -> Udcm/1
  Sum7/1 -> Uqcm/1
  We/1 -> Product1/1, ki3/1, Product/2
  ki3/1 -> Sum7/2
  Product/1 -> Sum7/1
  ki4/1 -> Product/1

== system Mains/Controller/Cur. Ctrl/Close i-Ctrl/PI(d) ==
  Eid : Inport
  (+-Uidm) : DiscreteIntegrator  SampleTime=Tsi  LimitOutput=on  UpperSaturationLimit=Uidm  LowerSaturationLimit=-Uidm  ICPrevOutput=DiscIntNeverNeededParam  ICPrevScaledInput=DiscIntNeverNeededParam
  Sum3 : Sum  SaturateOnIntegerOverflow=on  InputSameDT=on  OutDataTypeStr=Inherit: Same as first input
  ki1 : Gain  Gain=Ldo  SaturateOnIntegerOverflow=on  OutDataTypeStr=Inherit: Same as input  ParamDataTypeStr=Inherit: Same as input
  ki3 : Gain  Gain=Kid  SaturateOnIntegerOverflow=on  OutDataTypeStr=Inherit: Same as input  ParamDataTypeStr=Inherit: Same as input
  ki4 : Gain  Gain=1/Tid  SaturateOnIntegerOverflow=on  OutDataTypeStr=Inherit: Same as input  ParamDataTypeStr=Inherit: Same as input
  Ud* : Outport
  wires:
  ki3/1 -> ki1/1
  Sum3/1 -> Ud*/1
  ki4/1 -> (+-Uidm)/1
  Eid/1 -> ki3/1
  ki1/1 -> Sum3/1, ki4/1
  (+-Uidm)/1 -> Sum3/2

== system Mains/Controller/Cur. Ctrl/Close i-Ctrl/PI(q) ==
  Eiq : Inport
  (+-Uiqm) : DiscreteIntegrator  SampleTime=Tsi  LimitOutput=on  UpperSaturationLimit=Uiqm  LowerSaturationLimit=-Uiqm  ICPrevOutput=DiscIntNeverNeededParam  ICPrevScaledInput=DiscIntNeverNeededParam
  Sum3 : Sum  SaturateOnIntegerOverflow=on  InputSameDT=on  OutDataTypeStr=Inherit: Same as first input
  ki1 : Gain  Gain=Lqo  SaturateOnIntegerOverflow=on  OutDataTypeStr=Inherit: Same as input  ParamDataTypeStr=Inherit: Same as input
  ki3 : Gain  Gain=Kiq  SaturateOnIntegerOverflow=on  OutDataTypeStr=Inherit: Same as input  ParamDataTypeStr=Inherit: Same as input
  ki4 : Gain  Gain=1/Tiq  SaturateOnIntegerOverflow=on  OutDataTypeStr=Inherit: Same as input  ParamDataTypeStr=Inherit: Same as input
  Ud* : Outport
  wires:
  ki3/1 -> ki1/1
  Sum3/1 -> Ud*/1
  ki4/1 -> (+-Uiqm)/1
  Eiq/1 -> ki3/1
  ki1/1 -> Sum3/1, ki4/1
  (+-Uiqm)/1 -> Sum3/2

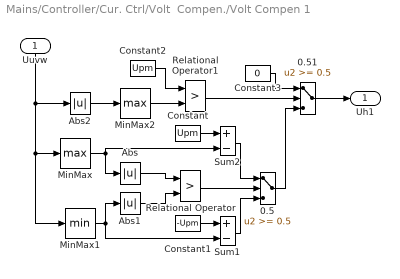
== system Mains/Controller/Cur. Ctrl/Volt  Compen./Volt Compen 1 ==
  Uuvw : Inport
  0.5 : Switch  Threshold=0.5  SaturateOnIntegerOverflow=on  InputSameDT=on
  0.51 : Switch  Threshold=0.5  SaturateOnIntegerOverflow=on  InputSameDT=on
  Abs : Abs  SaturateOnIntegerOverflow=on
  Abs1 : Abs  SaturateOnIntegerOverflow=on
  Abs2 : Abs  SaturateOnIntegerOverflow=on
  Constant : Constant  Value=Upm
  Constant1 : Constant  Value=-Upm
  Constant2 : Constant  Value=Upm
  Constant3 : Constant  Value=0
  MinMax : MinMax  Function=max  SaturateOnIntegerOverflow=on  InputSameDT=on
  MinMax1 : MinMax  SaturateOnIntegerOverflow=on  InputSameDT=on
  MinMax2 : MinMax  Function=max  SaturateOnIntegerOverflow=on  InputSameDT=on
  Relational Operator : RelationalOperator  Operator=>  InputSameDT=on
  Relational Operator1 : RelationalOperator  Operator=>  InputSameDT=on
  Sum1 : Sum  Inputs=+-  SaturateOnIntegerOverflow=on  InputSameDT=on  OutDataTypeStr=Inherit: Same as first input
  Sum2 : Sum  Inputs=+-  SaturateOnIntegerOverflow=on  InputSameDT=on  OutDataTypeStr=Inherit: Same as first input
  Uh1 : Outport
  wires:
  Constant3/1 -> 0.51/1
  0.51/1 -> Uh1/1
  Constant2/1 -> Relational Operator1/1
  MinMax2/1 -> Relational Operator1/2
  Relational Operator1/1 -> 0.51/2
  0.5/1 -> 0.51/3
  Abs2/1 -> MinMax2/1
  Uuvw/1 -> Abs2/1, MinMax1/1, MinMax/1
  Sum1/1 -> 0.5/3
  Sum2/1 -> 0.5/1
  Relational Operator/1 -> 0.5/2
  Abs1/1 -> Relational Operator/2
  Abs/1 -> Relational Operator/1
  MinMax1/1 -> Abs1/1, Sum1/2
  MinMax/1 -> Abs/1, Sum2/2
  Constant1/1 -> Sum1/1
  Constant/1 -> Sum2/1

== system Mains/Controller/Cur. Ctrl/Volt  Compen./Volt Compen 2 ==
  Uuvw : Inport
  MinMax : MinMax  Function=max  SaturateOnIntegerOverflow=on  InputSameDT=on
  MinMax1 : MinMax  SaturateOnIntegerOverflow=on  InputSameDT=on
  Sum3 : Sum  SaturateOnIntegerOverflow=on  InputSameDT=on  OutDataTypeStr=Inherit: Same as first input
  ki4 : Gain  Gain=-1/2  SaturateOnIntegerOverflow=on  OutDataTypeStr=Inherit: Same as input  ParamDataTypeStr=Inherit: Same as input
  Uh2 : Outport
  wires:
  ki4/1 -> Uh2/1
  MinMax/1 -> Sum3/1
  MinMax1/1 -> Sum3/2
  Uuvw/1 -> MinMax/1, MinMax1/1
  Sum3/1 -> ki4/1

== system Mains/Controller/Cur. Ctrl/fied weeking/PI(d) ==
  u_err : Inport
  integral up limit : Inport  Port=2
  integral down limit : Inport  Port=3
  output  up limit : Inport  Port=4
  output  down  limit : Inport  Port=5
  Discrete-Time Integrator : DiscreteIntegrator  InitialConditionSetting=State (most efficient)  ICPrevOutput=DiscIntNeverNeededParam  ICPrevScaledInput=DiscIntNeverNeededParam
  Saturation Dynamic : simulink/Discontinuities/Saturation Dynamic  OutMin=[]  OutMax=[]  OutDataTypeStr=Inherit: Same as second input  OutDataType=fixdt(1, 16)  OutScaling=2^-10  DoSatur=off
  Saturation Dynamic1 : simulink/Discontinuities/Saturation Dynamic  OutMin=[]  OutMax=[]  OutDataTypeStr=Inherit: Same as second input  OutDataType=fixdt(1, 16)  OutScaling=2^-10  DoSatur=off
  Sum3 : Sum  SaturateOnIntegerOverflow=on  InputSameDT=on  OutDataTypeStr=Inherit: Same as first input
  ki3 : Gain  Gain=fw_kp  SaturateOnIntegerOverflow=on  OutDataTypeStr=Inherit: Same as input  ParamDataTypeStr=Inherit: Same as input
  ki4 : Gain  Gain=fw_ki  SaturateOnIntegerOverflow=on  OutDataTypeStr=Inherit: Same as input  ParamDataTypeStr=Inherit: Same as input
  idc : Outport
  wires:
  u_err/1 -> ki3/1
  ki3/1 -> Sum3/1, ki4/1
  Saturation Dynamic/1 -> Sum3/2
  integral up limit/1 -> Saturation Dynamic/1
  integral down limit/1 -> Saturation Dynamic/3
  Saturation Dynamic1/1 -> idc/1
  Sum3/1 -> Saturation Dynamic1/2
  output  up limit/1 -> Saturation Dynamic1/1
  output  down  limit/1 -> Saturation Dynamic1/3
  ki4/1 -> Discrete-Time Integrator/1
  Discrete-Time Integrator/1 -> Saturation Dynamic/2

== system Mains/Controller/Cur. Ctrl/fied weeking/Tf(Ts) ==
  In1 : Inport
  LPF : DiscreteFilter  Numerator=[Ts/(Ts+TL)]  Denominator=[1 -(1-Ts/(Ts+TL))]  SampleTime=Ts
  Out1 : Outport
  wires:
  LPF/1 -> Out1/1
  In1/1 -> LPF/1

== system Mains/Controller/Cur. Ctrl/fied weeking/Tf(Ts)1 ==
  In1 : Inport
  LPF : DiscreteFilter  Numerator=[Ts/(Ts+TL)]  Denominator=[1 -(1-Ts/(Ts+TL))]  SampleTime=Ts
  Out1 : Outport
  wires:
  In1/1 -> LPF/1
  LPF/1 -> Out1/1

== system Mains/Controller/Cur. Ctrl/Close i-Ctrl/+-Urm1/Recalculate ==
  Ud/q : Inport
  Ur : Inport  Port=2
  Enable : EnablePort
  Constant : Constant  Value=Urm
  Product : Product  Inputs=**/  SaturateOnIntegerOverflow=on  InputSameDT=on  OutDataTypeStr=Inherit: Same as first input
  Tsi : ZeroOrderHold  SampleTime=Tsi
  Ud/qO : Outport
  wires:
  Ud/q/1 -> Product/1
  Product/1 -> Ud/qO/1
  Ur/1 -> Product/3
  Constant/1 -> Tsi/1
  Tsi/1 -> Product/2
